simulink model "Test_mcb_pmsm_foc_sim_RL"  (R2020b)
settings: Solver=FixedStepDiscrete  StartTime=0.0  StopTime=6  RelTol=1e-3  EnableMultiTasking=on
values from neighbouring files (symbols this model uses):
  coeff_d = readmatrix('C:\Users\terzo\LearningX\advanced_ML\model_tree\output_d\coeff.txt')    [readtrees.m]
  coeff_q = readmatrix('C:\Users\terzo\LearningX\advanced_ML\model_tree\output_q\coeff.txt')    [readtrees.m]
  index_d = readmatrix('C:\Users\terzo\LearningX\advanced_ML\model_tree\output_d\index.txt')    [readtrees.m]
  index_q = readmatrix('C:\Users\terzo\LearningX\advanced_ML\model_tree\output_q\index.txt')    [readtrees.m]
  intercept_d = readmatrix('C:\Users\terzo\LearningX\advanced_ML\model_tree\output_d\intercept.txt')    [readtrees.m]
  intercept_q = readmatrix('C:\Users\terzo\LearningX\advanced_ML\model_tree\output_q\intercept.txt')    [readtrees.m]
  inverter = mcb_SetInverterParameters_RL('BoostXL-DRV8305')    [sim_data.m]
  maxAngleIn = 1    [sim_data.m]
  MechOfstInputType = pmsm.p    [sim_data.m]
  PI_params = mcb.internal.SetControllerParameters(pmsm,inverter,PU_System,T_pwm,Ts,Ts_speed)    [sim_data.m]
  PU_System = mcb_SetPUSystem_RL(pmsm,inverter)    [sim_data.m]
  threshold_d = readmatrix('C:\Users\terzo\LearningX\advanced_ML\model_tree\output_d\treshold.txt')    [readtrees.m]
  threshold_q = readmatrix('C:\Users\terzo\LearningX\advanced_ML\model_tree\output_q\treshold.txt')    [readtrees.m]
  Ts_motor = T_pwm/2    (= 0.0001)    [sim_data.m]
  Ts_simulink = T_pwm/2    (= 0.0001)    [sim_data.m]
  Ts_speed = 10*Ts    (= 0.002)    [sim_data.m]
undefined symbols (not defined in the file or in its folder): DiscIntNeverNeededParam, pmsm
libraries: mcbcontrolslib x22, mcbpositiondecoderlib x6, simulink x4, mcbplantlib x2, autolibpmsmexterior x2, rllib x1
(part 1 of 2)
settings Model: ExtModeTrigDuration=8  Creator=The MathWorks, Inc.  LastModifiedBy=terzo
settings DataIOCC: DSMLogging=off  InspectSignalLogs=on
settings OptimizationCC: DefaultParameterBehavior=Inlined  DefaultUnderspecifiedDataType=single  EnhancedBackFolding=on  PassReuseOutputArgsAs=Individual arguments  ZeroExternalMemoryAtStartup=off  ZeroInternalMemoryAtStartup=off  MaxStackSize=1024  OptimizeBlockOrder=speed  DifferentSizesBufferReuse=on  OptimizationCustomize=off  DenormalBehavior=FlushToZero  EfficientTunableParamExpr=on
settings DebuggingCC: ParameterPrecisionLossMsg=none  ParameterTunabilityLossMsg=error
settings SFSimCC: MATLABDynamicMemAlloc=off  SimTargetLang=C++
settings RTWCC: Description=Embedded Coder  SystemTargetFile=ert.tlc  TemplateMakefile=ert_default_tmf  Toolchain=Texas Instruments Code Composer Studio (C2000)  TargetLang=C++
settings CodeAppCC: ForceParamTrailComments=on  IgnoreCustomStorageClasses=off  OperatorAnnotations=on  SimulinkDataObjDesc=on  SFDataObjDesc=on  InsertBlockDesc=on
settings ERTTargetCC: TargetLangStandard=C++03 (ISO)  CodeReplacementLibrary=TI C28x  CodeInterfacePackaging=C++ class  ExtModeStaticAllocSize=10000  RootIOFormat=Structure reference  ERTCustomFileTemplate=example_file_process.tlc

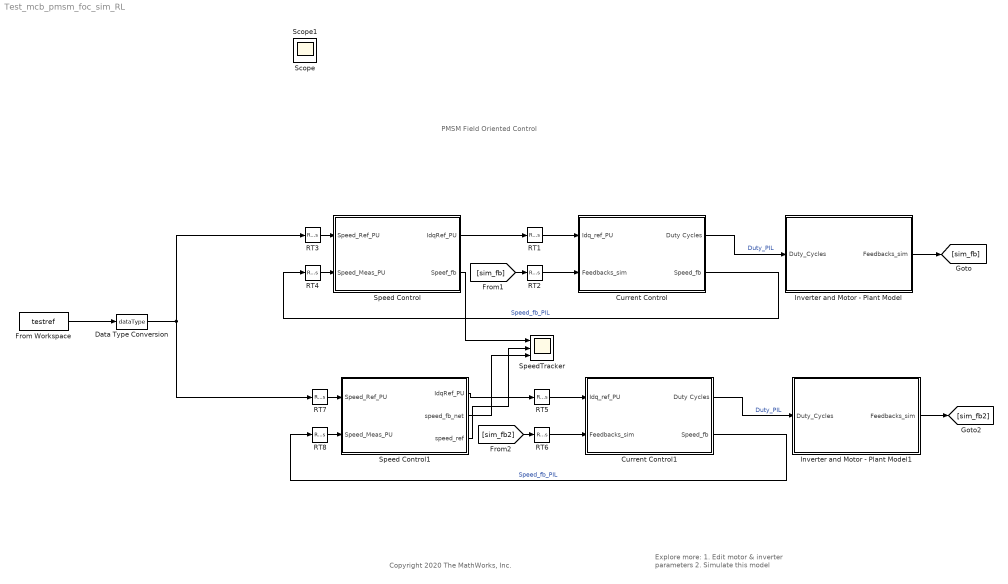
== system Test_mcb_pmsm_foc_sim_RL ==
  note: Explore more:
      | 1. Edit motor & inverter parameters
      | 2. Simulate this model
  note: PMSM Field Oriented Control
  note: Copyright 2020 The MathWorks, Inc.
  Current Control : Subsystem  TreatAsAtomicUnit=on
  Current Control1 : Subsystem  TreatAsAtomicUnit=on
  Data Type Conversion : DataTypeConversion  OutDataTypeStr=dataType
  From Workspace : FromWorkspace  VariableName=testref  SampleTime=Ts_speed
  Inverter and Motor - Plant Model : Subsystem
  Inverter and Motor - Plant Model1 : Subsystem
  RT{1..2,5..6} (4 alike) : RateTransition  Integrity=off  Deterministic=off  OutPortSampleTime=Ts
  RT{3..4,7..8} (4 alike) : RateTransition  Integrity=off  Deterministic=off  OutPortSampleTime=Ts_speed
  Speed Control : Subsystem  TreatAsAtomicUnit=on  SystemSampleTime=Ts_speed
  Speed Control1 : Subsystem  TreatAsAtomicUnit=on  SystemSampleTime=Ts_speed
  SpeedTracker : Scope  NumInputPorts=3
  Scope : Scope
  Scope1 : Scope
  wires:
  RT1/1 -> Current Control/1(Idq_ref_PU)
  Current Control/1(Duty Cycles) -> Inverter and Motor - Plant Model/1(Duty_Cycles)  "Duty_PIL"
  RT4/1 -> Speed Control/2(Speed_Meas_PU)
  Current Control/2(Speed_fb) -> RT4/1  "Speed_fb_PIL"
  [sim_fb] -> RT2/1
  Inverter and Motor - Plant Model/1(Feedbacks_sim) -> [sim_fb]
  RT3/1 -> Speed Control/1(Speed_Ref_PU)
  RT2/1 -> Current Control/2(Feedbacks_sim)
  Speed Control/1(IdqRef_PU) -> RT1/1
  From Workspace/1 -> Data Type Conversion/1
  RT7/1 -> Speed Control1/1(Speed_Ref_PU)
  Inverter and Motor - Plant Model1/1(Feedbacks_sim) -> [sim_fb2]
  RT6/1 -> Current Control1/2(Feedbacks_sim)
  Current Control1/1(Duty Cycles) -> Inverter and Motor - Plant Model1/1(Duty_Cycles)  "Duty_PIL"
  Speed Control1/1(IdqRef_PU) -> RT5/1
  Data Type Conversion/1 -> RT7/1, RT3/1
  RT5/1 -> Current Control1/1(Idq_ref_PU)
  [sim_fb2] -> RT6/1
  Current Control1/2(Speed_fb) -> RT8/1  "Speed_fb_PIL"
  RT8/1 -> Speed Control1/2(Speed_Meas_PU)
  Speed Control/2(Speef_fb) -> SpeedTracker/1
  Speed Control1/2(speed_fb_net) -> SpeedTracker/3
  Speed Control1/3(speed_ref) -> SpeedTracker/2

== system Test_mcb_pmsm_foc_sim_RL/Current Control ==
  Idq_ref_PU : Inport
  Feedbacks_sim : Inport  Port=2
  Control_System : Subsystem
  Demux1 : Demux
  Input Scaling : Subsystem
  Duty Cycles : Outport  InitialOutput=0  VectorParamsAs1DForOutWhenUnconnected=off
  Speed_fb : Outport  Port=2  InitialOutput=0  VectorParamsAs1DForOutWhenUnconnected=off
  wires:
  Input Scaling/2(Pos_PU) -> Control_System/2(Pos_PU)  "Pos_PU"
  Input Scaling/3(speed_PU) -> Speed_fb/1  "Speed_PU"
  Input Scaling/1(Iab_meas_PU) -> Control_System/1(Iab_meas_PU)  "Iab_fb_PU"
  Demux1/1 -> Input Scaling/1(Ia_ADC)
  Demux1/2 -> Input Scaling/2(Ib_ADC)
  Demux1/3 -> Input Scaling/3(QEP_Position_Count)
  Demux1/4 -> Input Scaling/4(QEP_Index_Latch)
  Control_System/1(Duty_Cycles) -> Duty Cycles/1
  Feedbacks_sim/1 -> Demux1/1
  Idq_ref_PU/1 -> Control_System/3(Idq_ref_PU)

== system Test_mcb_pmsm_foc_sim_RL/Current Control1 ==
  Idq_ref_PU : Inport
  Feedbacks_sim : Inport  Port=2
  Control_System : Subsystem
  Demux1 : Demux
  Input Scaling : Subsystem
  Duty Cycles : Outport  InitialOutput=0  VectorParamsAs1DForOutWhenUnconnected=off
  Speed_fb : Outport  Port=2  InitialOutput=0  VectorParamsAs1DForOutWhenUnconnected=off
  wires:
  Input Scaling/2(Pos_PU) -> Control_System/2(Pos_PU)  "Pos_PU"
  Input Scaling/3(speed_PU) -> Speed_fb/1  "Speed_PU"
  Input Scaling/1(Iab_meas_PU) -> Control_System/1(Iab_meas_PU)  "Iab_fb_PU"
  Demux1/1 -> Input Scaling/1(Ia_ADC)
  Demux1/2 -> Input Scaling/2(Ib_ADC)
  Demux1/3 -> Input Scaling/3(QEP_Position_Count)
  Demux1/4 -> Input Scaling/4(QEP_Index_Latch)
  Control_System/1(Duty_Cycles) -> Duty Cycles/1
  Feedbacks_sim/1 -> Demux1/1
  Idq_ref_PU/1 -> Control_System/3(Idq_ref_PU)

== system Test_mcb_pmsm_foc_sim_RL/Inverter and Motor - Plant Model ==
  Duty_Cycles : Inport
  Average Inverter : Subsystem
  Load_Profile (Torque) : Subsystem
  RT1 : RateTransition  Deterministic=off  OutPortSampleTime=Ts_simulink
  RT3 : RateTransition  Deterministic=off  OutPortSampleTime=Ts_simulink
  Rate Transition : RateTransition  Deterministic=off  OutPortSampleTime=Ts_motor
  Rate Transition1 : RateTransition  Deterministic=off  OutPortSampleTime=Ts_motor
  Sensor_Measurements : Subsystem
  Surface Mount PMSM : autolibpmsmexterior/Surface Mount PMSM  port_config=Torque  sim_type=Discrete  Ts=Ts_motor  FilePath=E:\Sandbox\Bauto\Work\surfacepmsm_motordata.m  P=pmsm.p  Rs=pmsm.Rs  Ldq_=pmsm.Ld  KConstText=Permanent flux linkage constant (lambda_pm):  lambda_pm=pmsm.FluxPM  Ke=159.9771  Kt=1.323  mechanical=[pmsm.J, pmsm.B, 0]  idq0=[0 0]  theta_init=0  omega_init=0  KConst=pmsm.FluxPM  lambda_pm_calc=pmsm.FluxPM  RefBlkName='autolibpmsmexterior/Surface Mount PMSM'  aMode=5  Ldq="[0.0002      0.0002]"
      settings: SourceProductBaseCode=PW,MT,UV,VE,VP
  Terminator : Terminator
  Feedbacks_sim : Outport  VectorParamsAs1DForOutWhenUnconnected=off
  wires:
  Surface Mount PMSM/1 -> RT3/1
  RT1/1 -> Sensor_Measurements/2(PhaseCurr)
  RT3/1 -> Sensor_Measurements/1(Info)
  Average Inverter/1(Vabc) -> Rate Transition/1
  Rate Transition/1 -> Surface Mount PMSM/2
  Surface Mount PMSM/3 -> Terminator/1
  Rate Transition1/1 -> Surface Mount PMSM/1
  Sensor_Measurements/1(Sim_fb) -> Feedbacks_sim/1
  Surface Mount PMSM/2 -> RT1/1  "Iabc"
  Load_Profile (Torque)/1(Load_Trq) -> Rate Transition1/1
  Duty_Cycles/1 -> Average Inverter/1(Duty_abc)

== system Test_mcb_pmsm_foc_sim_RL/Inverter and Motor - Plant Model1 ==
  Duty_Cycles : Inport
  Average Inverter : Subsystem
  Load_Profile (Torque) : Subsystem
  RT1 : RateTransition  Deterministic=off  OutPortSampleTime=Ts_simulink
  RT3 : RateTransition  Deterministic=off  OutPortSampleTime=Ts_simulink
  Rate Transition : RateTransition  Deterministic=off  OutPortSampleTime=Ts_motor
  Rate Transition1 : RateTransition  Deterministic=off  OutPortSampleTime=Ts_motor
  Sensor_Measurements : Subsystem
  Surface Mount PMSM : autolibpmsmexterior/Surface Mount PMSM  port_config=Torque  sim_type=Discrete  Ts=Ts_motor  FilePath=E:\Sandbox\Bauto\Work\surfacepmsm_motordata.m  P=pmsm.p  Rs=pmsm.Rs  Ldq_=pmsm.Ld  KConstText=Permanent flux linkage constant (lambda_pm):  lambda_pm=pmsm.FluxPM  Ke=159.9771  Kt=1.323  mechanical=[pmsm.J, pmsm.B, 0]  idq0=[0 0]  theta_init=0  omega_init=0  KConst=pmsm.FluxPM  lambda_pm_calc=pmsm.FluxPM  RefBlkName='autolibpmsmexterior/Surface Mount PMSM'  aMode=5  Ldq="[0.0002      0.0002]"
      settings: SourceProductBaseCode=PW,MT,UV,VE,VP
  Terminator : Terminator
  Feedbacks_sim : Outport  VectorParamsAs1DForOutWhenUnconnected=off
  wires:
  Surface Mount PMSM/1 -> RT3/1
  RT1/1 -> Sensor_Measurements/2(PhaseCurr)
  RT3/1 -> Sensor_Measurements/1(Info)
  Average Inverter/1(Vabc) -> Rate Transition/1
  Rate Transition/1 -> Surface Mount PMSM/2
  Surface Mount PMSM/3 -> Terminator/1
  Rate Transition1/1 -> Surface Mount PMSM/1
  Sensor_Measurements/1(Sim_fb) -> Feedbacks_sim/1
  Surface Mount PMSM/2 -> RT1/1  "Iabc"
  Load_Profile (Torque)/1(Load_Trq) -> Rate Transition1/1
  Duty_Cycles/1 -> Average Inverter/1(Duty_abc)

== system Test_mcb_pmsm_foc_sim_RL/Speed Control ==
  Speed_Ref_PU : Inport
  Speed_Meas_PU : Inport  Port=2
  Gain3 : Gain  Gain=pmsm.N_base
  IIR Filter : mcbcontrolslib/IIR Filter  Filter_constant=0.1
      settings: SourceProductBaseCode=MT
  Id_ref : Constant  Value=0  OutDataTypeStr=dataType  SampleTime=Ts_speed
  Mux1 : Mux  Inputs=2
  PI_Controller_Speed : Subsystem
  IdqRef_PU : Outport  VectorParamsAs1DForOutWhenUnconnected=off
  Speef_fb : Outport  Port=2
  wires:
  Speed_Meas_PU/1 -> Gain3/1, PI_Controller_Speed/2(N_fb)  "Speed_fb"
  Id_ref/1 -> Mux1/1
  PI_Controller_Speed/1(Iq_ref) -> Mux1/2
  Mux1/1 -> IdqRef_PU/1
  Speed_Ref_PU/1 -> IIR Filter/1  "Speed_Ref"
  IIR Filter/1 -> PI_Controller_Speed/1(N_ref)  "Speed_Ref"
  Gain3/1 -> Speef_fb/1  "speed_fb_rpm"

== system Test_mcb_pmsm_foc_sim_RL/Speed Control1 ==
  Speed_Ref_PU : Inport
  Speed_Meas_PU : Inport  Port=2
  Gain1 : Gain  Gain=pmsm.N_base
  Gain3 : Gain  Gain=pmsm.N_base
  IIR Filter : mcbcontrolslib/IIR Filter  Filter_constant=0.1
      settings: SourceProductBaseCode=MT
  Id_ref : Constant  Value=0  OutDataTypeStr=dataType  SampleTime=Ts_speed
  Mux1 : Mux  Inputs=2
  PI_Controller_Speed : Subsystem
  IdqRef_PU : Outport  VectorParamsAs1DForOutWhenUnconnected=off
  speed_fb_net : Outport  Port=2
  speed_ref : Outport  Port=3
  wires:
  Speed_Meas_PU/1 -> Gain3/1, PI_Controller_Speed/2(N_fb)  "Speed_fb"
  Id_ref/1 -> Mux1/1
  PI_Controller_Speed/1(Iq_ref) -> Mux1/2
  Mux1/1 -> IdqRef_PU/1
  Speed_Ref_PU/1 -> IIR Filter/1  "Speed_Ref"
  IIR Filter/1 -> Gain1/1, PI_Controller_Speed/1(N_ref)  "Speed_Ref"
  Gain3/1 -> speed_fb_net/1  "speed_fb_net_rpm"
  Gain1/1 -> speed_ref/1  "speed_ref_rpm"

== system Test_mcb_pmsm_foc_sim_RL/Current Control/Control_System ==
  Iab_meas_PU : Inport
  Pos_PU : Inport  Port=2
  Idq_ref_PU : Inport  Port=3
  Closed Loop Control : Subsystem
  Duty_Cycles : Outport  VectorParamsAs1DForOutWhenUnconnected=off
  wires:
  Iab_meas_PU/1 -> Closed Loop Control/1(Iab_meas_PU)
  Pos_PU/1 -> Closed Loop Control/2(Pos_PU)
  Idq_ref_PU/1 -> Closed Loop Control/3(Idq_ref_PU)
  Closed Loop Control/1(Vabc in PU) -> Duty_Cycles/1

== system Test_mcb_pmsm_foc_sim_RL/Current Control/Input Scaling ==
  note: Current Measurements
  note: Position & Speed Measurements
  note: QEP
  Ia_ADC : Inport
  Ib_ADC : Inport  Port=2
  QEP_Position_Count : Inport  Port=3
  QEP_Index_Latch : Inport  Port=4
  " Calculate Position and Speed" : Subsystem
  Calculate Phase Currents : Subsystem
  IndexOffset : Constant  Value=pmsm.PositionOffset  OutDataTypeStr=dataType  SampleTime=-1
  Iab_meas_PU : Outport
  Pos_PU : Outport  Port=2
  speed_PU : Outport  Port=3
  wires:
  " Calculate Position and Speed"/2(speed) -> speed_PU/1
  Calculate Phase Currents/1(Iab_meas_PU) -> Iab_meas_PU/1  "Iab_fb_PU"
  QEP_Position_Count/1 -> " Calculate Position and Speed"/1(QEP_Position_Count)
  " Calculate Position and Speed"/1(Theta_e) -> Pos_PU/1
  Ia_ADC/1 -> Calculate Phase Currents/1(Ia_ADC)
  Ib_ADC/1 -> Calculate Phase Currents/2(Ib_ADC)
  QEP_Index_Latch/1 -> " Calculate Position and Speed"/2(QEP_Index_Latch)
  IndexOffset/1 -> " Calculate Position and Speed"/3(Offset)

== system Test_mcb_pmsm_foc_sim_RL/Current Control1/Control_System ==
  Iab_meas_PU : Inport
  Pos_PU : Inport  Port=2
  Idq_ref_PU : Inport  Port=3
  Closed Loop Control : Subsystem
  Duty_Cycles : Outport  VectorParamsAs1DForOutWhenUnconnected=off
  wires:
  Iab_meas_PU/1 -> Closed Loop Control/1(Iab_meas_PU)
  Pos_PU/1 -> Closed Loop Control/2(Pos_PU)
  Idq_ref_PU/1 -> Closed Loop Control/3(Idq_ref_PU)
  Closed Loop Control/1(Vabc in PU) -> Duty_Cycles/1

== system Test_mcb_pmsm_foc_sim_RL/Current Control1/Input Scaling ==
  note: Current Measurements
  note: Position & Speed Measurements
  note: QEP
  Ia_ADC : Inport
  Ib_ADC : Inport  Port=2
  QEP_Position_Count : Inport  Port=3
  QEP_Index_Latch : Inport  Port=4
  " Calculate Position and Speed" : Subsystem
  Calculate Phase Currents : Subsystem
  IndexOffset : Constant  Value=pmsm.PositionOffset  OutDataTypeStr=dataType  SampleTime=-1
  Iab_meas_PU : Outport
  Pos_PU : Outport  Port=2
  speed_PU : Outport  Port=3
  wires:
  " Calculate Position and Speed"/2(speed) -> speed_PU/1
  Calculate Phase Currents/1(Iab_meas_PU) -> Iab_meas_PU/1  "Iab_fb_PU"
  QEP_Position_Count/1 -> " Calculate Position and Speed"/1(QEP_Position_Count)
  " Calculate Position and Speed"/1(Theta_e) -> Pos_PU/1
  Ia_ADC/1 -> Calculate Phase Currents/1(Ia_ADC)
  Ib_ADC/1 -> Calculate Phase Currents/2(Ib_ADC)
  QEP_Index_Latch/1 -> " Calculate Position and Speed"/2(QEP_Index_Latch)
  IndexOffset/1 -> " Calculate Position and Speed"/3(Offset)

== system Test_mcb_pmsm_foc_sim_RL/Inverter and Motor - Plant Model/Average Inverter ==
  Duty_abc : Inport
  Average-Value Inverter : mcbplantlib/Average-Value Inverter
  Constant2 : Constant  Value=inverter.V_dc  OutDataTypeStr=single  SampleTime=-1
  Data Type Conversion1 : DataTypeConversion  OutDataTypeStr=single  RndMeth=Simplest
  Rate Transition3 : RateTransition  Deterministic=off  OutPortSampleTime=Ts_inverter
  Vabc : Outport  VectorParamsAs1DForOutWhenUnconnected=off
  wires:
  Constant2/1 -> Average-Value Inverter/2
  Data Type Conversion1/1 -> Rate Transition3/1
  Duty_abc/1 -> Data Type Conversion1/1
  Rate Transition3/1 -> Average-Value Inverter/1
  Average-Value Inverter/1 -> Vabc/1

== system Test_mcb_pmsm_foc_sim_RL/Inverter and Motor - Plant Model/Load_Profile (Torque) ==
  Data Type Conversion : DataTypeConversion  OutDataTypeStr=single
  IIR Filter : mcbcontrolslib/IIR Filter  Filter_constant=0.01
      settings: SourceProductBaseCode=MT
  T_load : Step  Time=100  After=0  SampleTime=Ts_simulink
  T_load1 : Step  Commented=on  Time=0.8  Before=0.05*pmsm.T_rated  After=0.05*pmsm.T_rated  SampleTime=Ts_simulink
  Load_Trq : Outport  VectorParamsAs1DForOutWhenUnconnected=off
  wires:
  Data Type Conversion/1 -> IIR Filter/1
  IIR Filter/1 -> Load_Trq/1
  T_load/1 -> Data Type Conversion/1

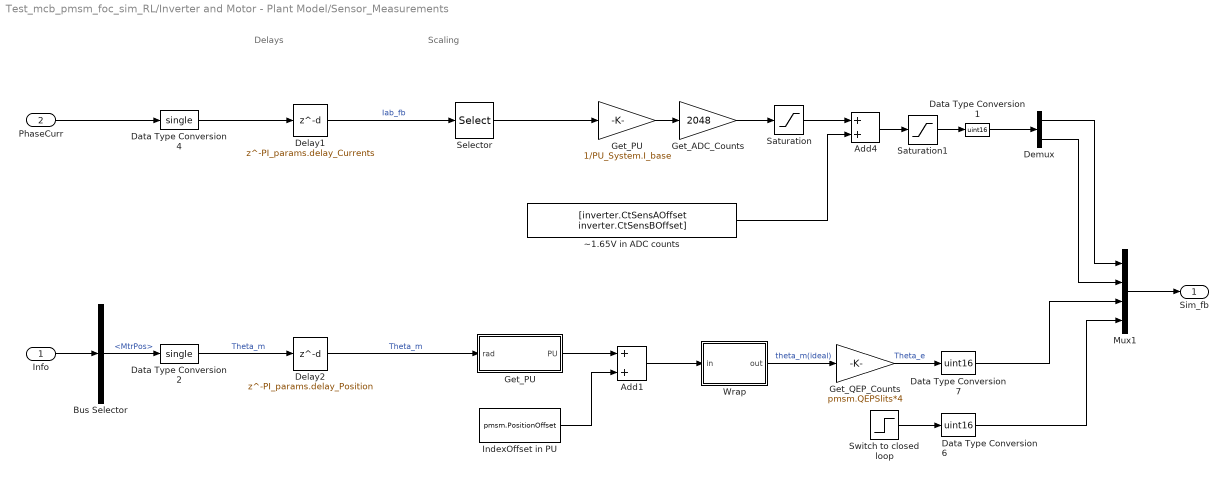
== system Test_mcb_pmsm_foc_sim_RL/Inverter and Motor - Plant Model/Sensor_Measurements ==
  note: Scaling
  note: Delays
  Info : Inport
  PhaseCurr : Inport  Port=2
  Add1 : Sum  RndMeth=Simplest
  Add4 : Sum  OutDataTypeStr=uint16
  Bus Selector : BusSelector  OutputSignals=MtrPos
  Data Type Conversion1 : DataTypeConversion  OutDataTypeStr=uint16
  Data Type Conversion2 : DataTypeConversion  OutDataTypeStr=single  RndMeth=Simplest
  Data Type Conversion4 : DataTypeConversion  OutDataTypeStr=single  RndMeth=Simplest
  Data Type Conversion6 : DataTypeConversion  OutDataTypeStr=uint16  RndMeth=Simplest
  Data Type Conversion7 : DataTypeConversion  OutDataTypeStr=uint16  RndMeth=Simplest
  Delay1 : Delay  DelayLength=PI_params.delay_Currents
  Delay2 : Delay  DelayLength=PI_params.delay_Position
  Demux : Demux  Outputs=2
  Get_ADC_Counts : Gain  Gain=2048  RndMeth=Simplest  OutDataTypeStr=Inherit: Same as input
  Get_PU : Gain  Gain=1/PU_System.I_base  RndMeth=Simplest
  "Get_PU " : Subsystem
  Get_QEP_Counts : Gain  Gain=pmsm.QEPSlits*4  OutDataTypeStr=uint16  RndMeth=Simplest
  IndexOffset in PU : Constant  Value=pmsm.PositionOffset  OutDataTypeStr=single  SampleTime=-1
  Mux1 : Mux
  Saturation : Saturate  UpperLimit=2048  LowerLimit=-2048
  Saturation1 : Saturate  UpperLimit=4095  LowerLimit=0
  Selector : Selector  InputPortWidth=3  IndexOptions=Index vector (dialog)  Indices=[1 2]  OutputSizes=1
  "Switch to closed loop " : Step  Time=0.1  SampleTime=Ts_motor
  Wrap : Subsystem
  ~1.65V in ADC counts : Constant  Value=[inverter.CtSensAOffset inverter.CtSensBOffset]  OutDataTypeStr=uint16  SampleTime=-1
  Sim_fb : Outport  VectorParamsAs1DForOutWhenUnconnected=off
  wires:
  Get_ADC_Counts/1 -> Saturation/1
  Saturation1/1 -> Data Type Conversion1/1
  Add4/1 -> Saturation1/1
  Data Type Conversion1/1 -> Demux/1
  ~1.65V in ADC counts/1 -> Add4/2
  Delay1/1 -> Selector/1  "Iab_fb"
  Saturation/1 -> Add4/1
  Data Type Conversion4/1 -> Delay1/1
  Selector/1 -> Get_PU/1
  PhaseCurr/1 -> Data Type Conversion4/1
  Get_PU/1 -> Get_ADC_Counts/1
  Info/1 -> Bus Selector/1
  Bus Selector/1 -> Data Type Conversion2/1  "<MtrPos>"
  Demux/1 -> Mux1/1
  Mux1/1 -> Sim_fb/1
  Demux/2 -> Mux1/2
  Data Type Conversion2/1 -> Delay2/1  "Theta_m"
  Add1/1 -> Wrap/1(in)
  Delay2/1 -> "Get_PU "/1(rad)  "Theta_m"
  Wrap/1(out) -> Get_QEP_Counts/1  "theta_m(ideal)"
  "Get_PU "/1(PU) -> Add1/1
  Get_QEP_Counts/1 -> Data Type Conversion7/1  "Theta_e"
  IndexOffset in PU/1 -> Add1/2
  Data Type Conversion7/1 -> Mux1/3
  Data Type Conversion6/1 -> Mux1/4
  "Switch to closed loop "/1 -> Data Type Conversion6/1

== system Test_mcb_pmsm_foc_sim_RL/Inverter and Motor - Plant Model1/Average Inverter ==
  Duty_abc : Inport
  Average-Value Inverter : mcbplantlib/Average-Value Inverter
  Constant2 : Constant  Value=inverter.V_dc  OutDataTypeStr=single  SampleTime=-1
  Data Type Conversion1 : DataTypeConversion  OutDataTypeStr=single  RndMeth=Simplest
  Rate Transition3 : RateTransition  Deterministic=off  OutPortSampleTime=Ts_inverter
  Vabc : Outport  VectorParamsAs1DForOutWhenUnconnected=off
  wires:
  Constant2/1 -> Average-Value Inverter/2
  Data Type Conversion1/1 -> Rate Transition3/1
  Duty_abc/1 -> Data Type Conversion1/1
  Rate Transition3/1 -> Average-Value Inverter/1
  Average-Value Inverter/1 -> Vabc/1

== system Test_mcb_pmsm_foc_sim_RL/Inverter and Motor - Plant Model1/Load_Profile (Torque) ==
  Data Type Conversion : DataTypeConversion  OutDataTypeStr=single
  IIR Filter : mcbcontrolslib/IIR Filter  Filter_constant=0.01
      settings: SourceProductBaseCode=MT
  T_load : Step  Time=100  After=0  SampleTime=Ts_simulink
  T_load1 : Step  Commented=on  Time=0.8  Before=0.05*pmsm.T_rated  After=0.05*pmsm.T_rated  SampleTime=Ts_simulink
  Load_Trq : Outport  VectorParamsAs1DForOutWhenUnconnected=off
  wires:
  Data Type Conversion/1 -> IIR Filter/1
  IIR Filter/1 -> Load_Trq/1
  T_load/1 -> Data Type Conversion/1

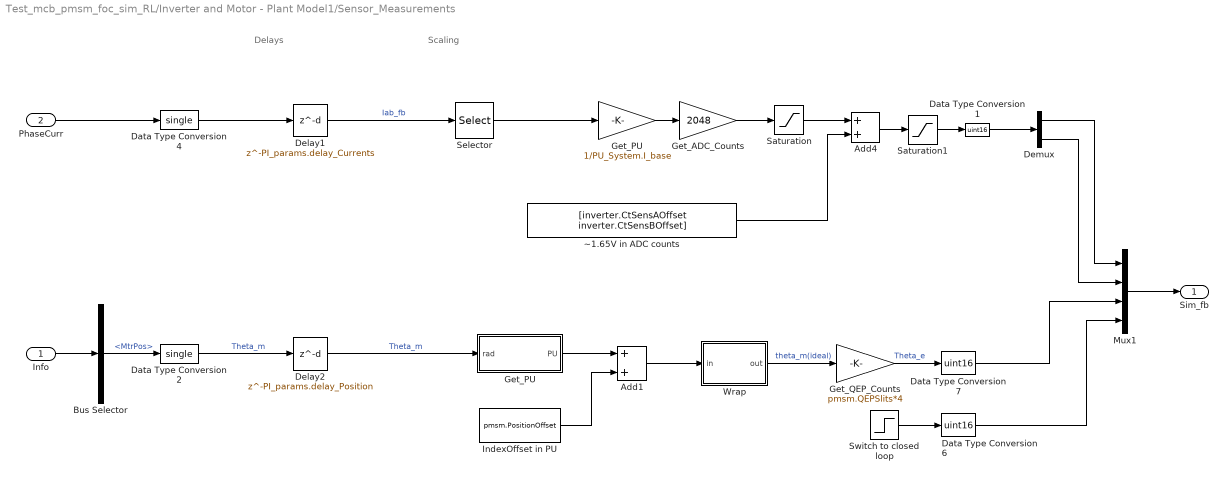
== system Test_mcb_pmsm_foc_sim_RL/Inverter and Motor - Plant Model1/Sensor_Measurements ==
  note: Scaling
  note: Delays
  Info : Inport
  PhaseCurr : Inport  Port=2
  Add1 : Sum  RndMeth=Simplest
  Add4 : Sum  OutDataTypeStr=uint16
  Bus Selector : BusSelector  OutputSignals=MtrPos
  Data Type Conversion1 : DataTypeConversion  OutDataTypeStr=uint16
  Data Type Conversion2 : DataTypeConversion  OutDataTypeStr=single  RndMeth=Simplest
  Data Type Conversion4 : DataTypeConversion  OutDataTypeStr=single  RndMeth=Simplest
  Data Type Conversion6 : DataTypeConversion  OutDataTypeStr=uint16  RndMeth=Simplest
  Data Type Conversion7 : DataTypeConversion  OutDataTypeStr=uint16  RndMeth=Simplest
  Delay1 : Delay  DelayLength=PI_params.delay_Currents
  Delay2 : Delay  DelayLength=PI_params.delay_Position
  Demux : Demux  Outputs=2
  Get_ADC_Counts : Gain  Gain=2048  RndMeth=Simplest  OutDataTypeStr=Inherit: Same as input
  Get_PU : Gain  Gain=1/PU_System.I_base  RndMeth=Simplest
  "Get_PU " : Subsystem
  Get_QEP_Counts : Gain  Gain=pmsm.QEPSlits*4  OutDataTypeStr=uint16  RndMeth=Simplest
  IndexOffset in PU : Constant  Value=pmsm.PositionOffset  OutDataTypeStr=single  SampleTime=-1
  Mux1 : Mux
  Saturation : Saturate  UpperLimit=2048  LowerLimit=-2048
  Saturation1 : Saturate  UpperLimit=4095  LowerLimit=0
  Selector : Selector  InputPortWidth=3  IndexOptions=Index vector (dialog)  Indices=[1 2]  OutputSizes=1
  "Switch to closed loop " : Step  Time=0.1  SampleTime=Ts_motor
  Wrap : Subsystem
  ~1.65V in ADC counts : Constant  Value=[inverter.CtSensAOffset inverter.CtSensBOffset]  OutDataTypeStr=uint16  SampleTime=-1
  Sim_fb : Outport  VectorParamsAs1DForOutWhenUnconnected=off
  wires:
  Get_ADC_Counts/1 -> Saturation/1
  Saturation1/1 -> Data Type Conversion1/1
  Add4/1 -> Saturation1/1
  Data Type Conversion1/1 -> Demux/1
  ~1.65V in ADC counts/1 -> Add4/2
  Delay1/1 -> Selector/1  "Iab_fb"
  Saturation/1 -> Add4/1
  Data Type Conversion4/1 -> Delay1/1
  Selector/1 -> Get_PU/1
  PhaseCurr/1 -> Data Type Conversion4/1
  Get_PU/1 -> Get_ADC_Counts/1
  Info/1 -> Bus Selector/1
  Bus Selector/1 -> Data Type Conversion2/1  "<MtrPos>"
  Demux/1 -> Mux1/1
  Mux1/1 -> Sim_fb/1
  Demux/2 -> Mux1/2
  Data Type Conversion2/1 -> Delay2/1  "Theta_m"
  Add1/1 -> Wrap/1(in)
  Delay2/1 -> "Get_PU "/1(rad)  "Theta_m"
  Wrap/1(out) -> Get_QEP_Counts/1  "theta_m(ideal)"
  "Get_PU "/1(PU) -> Add1/1
  Get_QEP_Counts/1 -> Data Type Conversion7/1  "Theta_e"
  IndexOffset in PU/1 -> Add1/2
  Data Type Conversion7/1 -> Mux1/3
  Data Type Conversion6/1 -> Mux1/4
  "Switch to closed loop "/1 -> Data Type Conversion6/1

== system Test_mcb_pmsm_foc_sim_RL/Speed Control/PI_Controller_Speed ==
  N_ref : Inport
  N_fb : Inport  Port=2
  Constant : Constant  OutDataTypeStr=boolean
  Discrete PI Controller with anti-windup & reset : mcbcontrolslib/Discrete PI Controller  with anti-windup & reset  UpperSaturationLimit=1  LowerSaturationLimit=-1
      settings: SourceProductBaseCode=MT
  Ki1 : Constant  Value=PI_params.Ki_speed*Ts_speed  OutDataTypeStr=dataType  SampleTime=-1
  Ki2 : Constant  Value=0  OutDataTypeStr=dataType  SampleTime=-1
  Kp1 : Constant  Value=PI_params.Kp_speed  OutDataTypeStr=dataType  SampleTime=-1
  Logical Operator : Logic  Operator=NOT  IconShape=distinctive  AllPortsSameDT=off  OutDataTypeStr=boolean
  Sum : Sum  Inputs=|+-  OutDataTypeStr=Inherit: Same as first input
  Iq_ref : Outport  VectorParamsAs1DForOutWhenUnconnected=off
  wires:
  Discrete PI Controller with anti-windup & reset/1 -> Iq_ref/1
  Ki1/1 -> Discrete PI Controller with anti-windup & reset/3
  Kp1/1 -> Discrete PI Controller with anti-windup & reset/2
  N_fb/1 -> Sum/2
  N_ref/1 -> Sum/1
  Sum/1 -> Discrete PI Controller with anti-windup & reset/1
  Logical Operator/1 -> Discrete PI Controller with anti-windup & reset/4
  Ki2/1 -> Discrete PI Controller with anti-windup & reset/5
  Constant/1 -> Logical Operator/1

== system Test_mcb_pmsm_foc_sim_RL/Speed Control1/PI_Controller_Speed ==
  N_ref : Inport
  N_fb : Inport  Port=2
  Constant : Constant  OutDataTypeStr=boolean
  Discrete PI Controller with anti-windup & reset : mcbcontrolslib/Discrete PI Controller  with anti-windup & reset  UpperSaturationLimit=1  LowerSaturationLimit=-1
      settings: SourceProductBaseCode=MT
  Ki1 : Constant  Value=PI_params.Ki_speed*Ts_speed  OutDataTypeStr=dataType  SampleTime=-1
  Ki2 : Constant  Value=0  OutDataTypeStr=dataType  SampleTime=-1
  Kp1 : Constant  Value=PI_params.Kp_speed  OutDataTypeStr=dataType  SampleTime=-1
  Logical Operator : Logic  Operator=NOT  IconShape=distinctive  AllPortsSameDT=off  OutDataTypeStr=boolean
  Sum : Sum  Inputs=|+-  OutDataTypeStr=Inherit: Same as first input
  Iq_ref : Outport  VectorParamsAs1DForOutWhenUnconnected=off
  wires:
  Discrete PI Controller with anti-windup & reset/1 -> Iq_ref/1
  Ki1/1 -> Discrete PI Controller with anti-windup & reset/3
  Kp1/1 -> Discrete PI Controller with anti-windup & reset/2
  N_fb/1 -> Sum/2
  N_ref/1 -> Sum/1
  Sum/1 -> Discrete PI Controller with anti-windup & reset/1
  Logical Operator/1 -> Discrete PI Controller with anti-windup & reset/4
  Ki2/1 -> Discrete PI Controller with anti-windup & reset/5
  Constant/1 -> Logical Operator/1

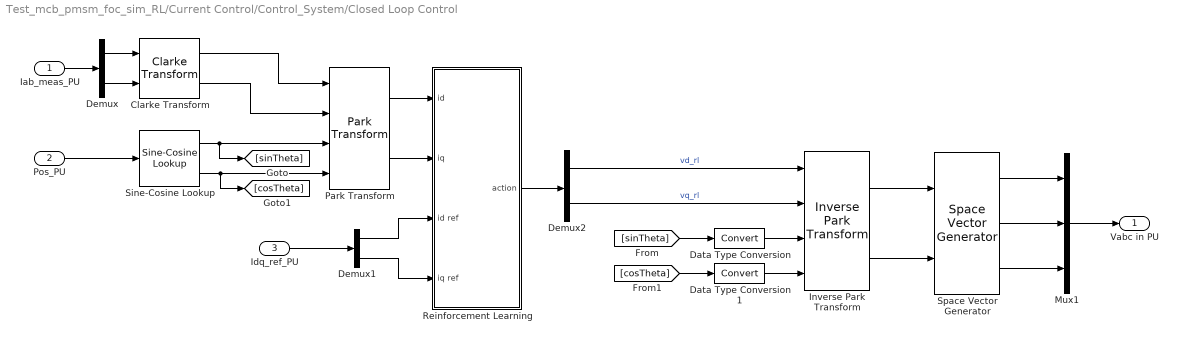
== system Test_mcb_pmsm_foc_sim_RL/Current Control/Control_System/Closed Loop Control ==
  Iab_meas_PU : Inport
  Pos_PU : Inport  Port=2
  Idq_ref_PU : Inport  Port=3
  Clarke Transform : mcbcontrolslib/Clarke Transform  VariantControl=Variant2
  Data Type Conversion : DataTypeConversion
  Data Type Conversion1 : DataTypeConversion
  Demux : Demux  Outputs=2
  Demux1 : Demux  Outputs=2
  Demux2 : Demux  Outputs=2
  Inverse Park Transform : mcbcontrolslib/Inverse Park Transform  AxisAlignment=D-axis
  Mux1 : Mux  Inputs=3
  Park Transform : mcbcontrolslib/Park Transform  AxisAlignment=D-axis
      settings: SourceProductBaseCode=MT
  Reinforcement Learning : Subsystem
  Sine-Cosine Lookup : mcbcontrolslib/Sine-Cosine Lookup  AngleInput=Per-unit  N_points=1024
      settings: SourceProductBaseCode=MT
  Space Vector Generator : mcbcontrolslib/Space Vector Generator
      settings: SourceProductBaseCode=MT
  Vabc in PU : Outport  VectorParamsAs1DForOutWhenUnconnected=off
  wires:
  Sine-Cosine Lookup/1 -> [sinTheta], Park Transform/3
  Clarke Transform/2 -> Park Transform/2
  Demux/2 -> Clarke Transform/2
  Pos_PU/1 -> Sine-Cosine Lookup/1
  Demux/1 -> Clarke Transform/1
  Inverse Park Transform/2 -> Space Vector Generator/2
  Iab_meas_PU/1 -> Demux/1
  Demux2/1 -> Inverse Park Transform/1  "vd_rl"
  Inverse Park Transform/1 -> Space Vector Generator/1
  Sine-Cosine Lookup/2 -> Park Transform/4, [cosTheta]
  Space Vector Generator/3 -> Mux1/3
  Demux2/2 -> Inverse Park Transform/2  "vq_rl"
  Space Vector Generator/1 -> Mux1/1
  Mux1/1 -> Vabc in PU/1
  Clarke Transform/1 -> Park Transform/1
  Space Vector Generator/2 -> Mux1/2
  Park Transform/1 -> Reinforcement Learning/1(id)
  Park Transform/2 -> Reinforcement Learning/2(iq)
  Idq_ref_PU/1 -> Demux1/1
  Demux1/1 -> Reinforcement Learning/3(id ref)
  Demux1/2 -> Reinforcement Learning/4(iq ref)
  Reinforcement Learning/1(action) -> Demux2/1
  [sinTheta] -> Data Type Conversion/1
  [cosTheta] -> Data Type Conversion1/1
  Data Type Conversion/1 -> Inverse Park Transform/3
  Data Type Conversion1/1 -> Inverse Park Transform/4

== system Test_mcb_pmsm_foc_sim_RL/Current Control/Input Scaling/ Calculate Position and Speed ==
  QEP_Position_Count : Inport
  QEP_Index_Latch : Inport  Port=2
  Offset : Inport  Port=3
  IIR Filter : mcbcontrolslib/IIR Filter  Filter_constant=0.01
      settings: SourceProductBaseCode=MT
  Mechanical to Electrical Position : mcbpositiondecoderlib/Mechanical to Electrical Position  Commented=on  NrPP=pmsm.p  selectedRange=Per unit  MechOfstInputType=Input port  mechOffsetIn=0  maxAngleIn=1  InputDataType=dataType  VariantSelect=fixed-point
      settings: SourceProductBaseCode=MT
  Quadrature Decoder : mcbpositiondecoderlib/Quadrature Decoder  EncoderSlitsPerRevolution=pmsm.QEPSlits  EncoderCountsPerSlit=4  CounterSize=16 bits  ExternalIndexCount=on  PositionUnit=Per unit  PositionDataType=dataType
      settings: SourceProductBaseCode=MT
  Speed Measurement : mcbpositiondecoderlib/Speed Measurement  PositionUnit=Per unit  SpeedCalculationMode=Time interval for speed calculation  SampleTimeAsync=Ts  MaximumApplicationSpeed=6000  SpeedResolution=5e-6  DelayLength=20  MaximumMeasurableSpeed=7499  MeasurableSpeedResolution=3.4925e-06  SpeedUnit=Per unit based on dialog  PerUnitSpeed=PU_System.N_base  SpeedDataType=dataType
      settings: SourceProductBaseCode=MT
  fixed-point : Subsystem  VariantControl=fixed-point
  Theta_e : Outport  VectorParamsAs1DForOutWhenUnconnected=off
  speed : Outport  Port=2  VectorParamsAs1DForOutWhenUnconnected=off
  wires:
  Speed Measurement/1 -> IIR Filter/1
  QEP_Position_Count/1 -> Quadrature Decoder/1
  Quadrature Decoder/1 -> fixed-point/1(ϴm), Speed Measurement/1
  Offset/1 -> fixed-point/2(Offset)
  IIR Filter/1 -> speed/1
  QEP_Index_Latch/1 -> Quadrature Decoder/2
  fixed-point/1(ϴe) -> Theta_e/1

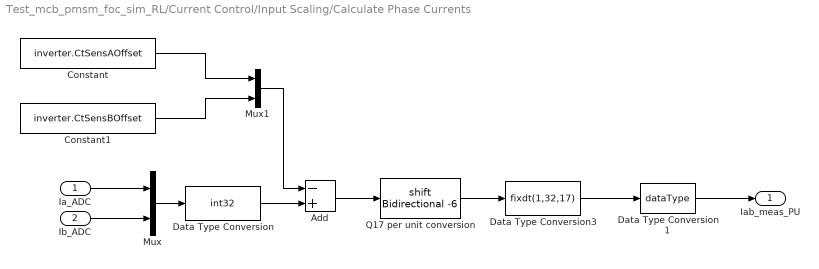
== system Test_mcb_pmsm_foc_sim_RL/Current Control/Input Scaling/Calculate Phase Currents ==
  Ia_ADC : Inport
  Ib_ADC : Inport  Port=2
  Add : Sum  Inputs=-+
  Constant : Constant  Value=inverter.CtSensAOffset  OutDataTypeStr=uint16
  Constant1 : Constant  Value=inverter.CtSensBOffset  OutDataTypeStr=uint16
  Data Type Conversion : DataTypeConversion  OutDataTypeStr=int32  ConvertRealWorld=Stored Integer (SI)  RndMeth=Simplest
  Data Type Conversion1 : DataTypeConversion  OutDataTypeStr=dataType  RndMeth=Simplest
  Data Type Conversion3 : DataTypeConversion  OutDataTypeStr=fixdt(1,32,17)  ConvertRealWorld=Stored Integer (SI)  RndMeth=Simplest
  Mux : Mux  Inputs=2
  Mux1 : Mux  Inputs=2
  Q17 per unit conversion : ArithShift  BitShiftNumber=-6
  Iab_meas_PU : Outport  VectorParamsAs1DForOutWhenUnconnected=off
  wires:
  Q17 per unit conversion/1 -> Data Type Conversion3/1
  Data Type Conversion/1 -> Add/2
  Add/1 -> Q17 per unit conversion/1
  Data Type Conversion3/1 -> Data Type Conversion1/1
  Data Type Conversion1/1 -> Iab_meas_PU/1
  Ia_ADC/1 -> Mux/1
  Ib_ADC/1 -> Mux/2
  Mux/1 -> Data Type Conversion/1
  Constant/1 -> Mux1/1
  Constant1/1 -> Mux1/2
  Mux1/1 -> Add/1

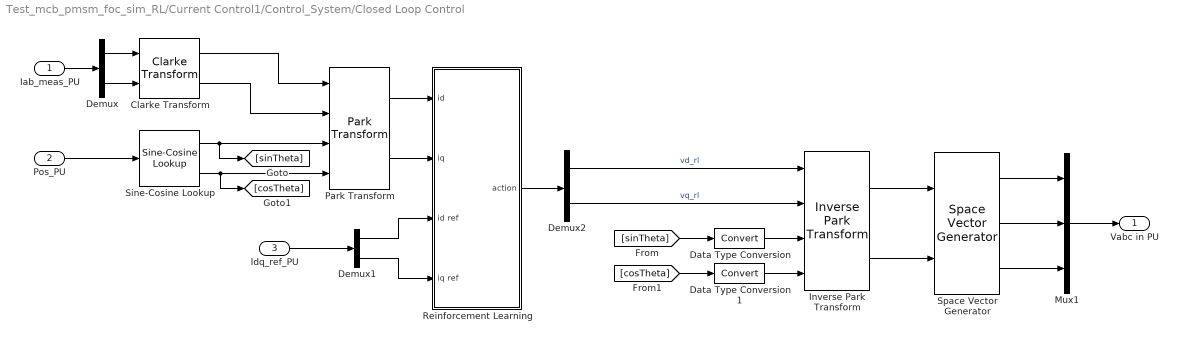
== system Test_mcb_pmsm_foc_sim_RL/Current Control1/Control_System/Closed Loop Control ==
  Iab_meas_PU : Inport
  Pos_PU : Inport  Port=2
  Idq_ref_PU : Inport  Port=3
  Clarke Transform : mcbcontrolslib/Clarke Transform  VariantControl=Variant2
  Data Type Conversion : DataTypeConversion
  Data Type Conversion1 : DataTypeConversion
  Demux : Demux  Outputs=2
  Demux1 : Demux  Outputs=2
  Demux2 : Demux  Outputs=2
  Inverse Park Transform : mcbcontrolslib/Inverse Park Transform  AxisAlignment=D-axis
  Mux1 : Mux  Inputs=3
  Park Transform : mcbcontrolslib/Park Transform  AxisAlignment=D-axis
      settings: SourceProductBaseCode=MT
  Reinforcement Learning : Subsystem
  Sine-Cosine Lookup : mcbcontrolslib/Sine-Cosine Lookup  AngleInput=Per-unit  N_points=1024
      settings: SourceProductBaseCode=MT
  Space Vector Generator : mcbcontrolslib/Space Vector Generator
      settings: SourceProductBaseCode=MT
  Vabc in PU : Outport  VectorParamsAs1DForOutWhenUnconnected=off
  wires:
  Sine-Cosine Lookup/1 -> [sinTheta], Park Transform/3
  Clarke Transform/2 -> Park Transform/2
  Demux/2 -> Clarke Transform/2
  Pos_PU/1 -> Sine-Cosine Lookup/1
  Demux/1 -> Clarke Transform/1
  Inverse Park Transform/2 -> Space Vector Generator/2
  Iab_meas_PU/1 -> Demux/1
  Demux2/1 -> Inverse Park Transform/1  "vd_rl"
  Inverse Park Transform/1 -> Space Vector Generator/1
  Sine-Cosine Lookup/2 -> Park Transform/4, [cosTheta]
  Space Vector Generator/3 -> Mux1/3
  Demux2/2 -> Inverse Park Transform/2  "vq_rl"
  Space Vector Generator/1 -> Mux1/1
  Mux1/1 -> Vabc in PU/1
  Clarke Transform/1 -> Park Transform/1
  Space Vector Generator/2 -> Mux1/2
  Park Transform/1 -> Reinforcement Learning/1(id)
  Park Transform/2 -> Reinforcement Learning/2(iq)
  Idq_ref_PU/1 -> Demux1/1
  Demux1/1 -> Reinforcement Learning/3(id ref)
  Demux1/2 -> Reinforcement Learning/4(iq ref)
  Reinforcement Learning/1(action) -> Demux2/1
  [sinTheta] -> Data Type Conversion/1
  [cosTheta] -> Data Type Conversion1/1
  Data Type Conversion/1 -> Inverse Park Transform/3
  Data Type Conversion1/1 -> Inverse Park Transform/4

== system Test_mcb_pmsm_foc_sim_RL/Current Control1/Input Scaling/ Calculate Position and Speed ==
  QEP_Position_Count : Inport
  QEP_Index_Latch : Inport  Port=2
  Offset : Inport  Port=3
  IIR Filter : mcbcontrolslib/IIR Filter  Filter_constant=0.01
      settings: SourceProductBaseCode=MT
  Mechanical to Electrical Position : mcbpositiondecoderlib/Mechanical to Electrical Position  Commented=on  NrPP=pmsm.p  selectedRange=Per unit  MechOfstInputType=Input port  mechOffsetIn=0  maxAngleIn=1  InputDataType=dataType  VariantSelect=fixed-point
      settings: SourceProductBaseCode=MT
  Quadrature Decoder : mcbpositiondecoderlib/Quadrature Decoder  EncoderSlitsPerRevolution=pmsm.QEPSlits  EncoderCountsPerSlit=4  CounterSize=16 bits  ExternalIndexCount=on  PositionUnit=Per unit  PositionDataType=dataType
      settings: SourceProductBaseCode=MT
  Speed Measurement : mcbpositiondecoderlib/Speed Measurement  PositionUnit=Per unit  SpeedCalculationMode=Time interval for speed calculation  SampleTimeAsync=Ts  MaximumApplicationSpeed=6000  SpeedResolution=5e-6  DelayLength=20  MaximumMeasurableSpeed=7499  MeasurableSpeedResolution=3.4925e-06  SpeedUnit=Per unit based on dialog  PerUnitSpeed=PU_System.N_base  SpeedDataType=dataType
      settings: SourceProductBaseCode=MT
  fixed-point : Subsystem  VariantControl=fixed-point
  Theta_e : Outport  VectorParamsAs1DForOutWhenUnconnected=off
  speed : Outport  Port=2  VectorParamsAs1DForOutWhenUnconnected=off
  wires:
  Speed Measurement/1 -> IIR Filter/1
  QEP_Position_Count/1 -> Quadrature Decoder/1
  Quadrature Decoder/1 -> fixed-point/1(ϴm), Speed Measurement/1
  Offset/1 -> fixed-point/2(Offset)
  IIR Filter/1 -> speed/1
  QEP_Index_Latch/1 -> Quadrature Decoder/2
  fixed-point/1(ϴe) -> Theta_e/1

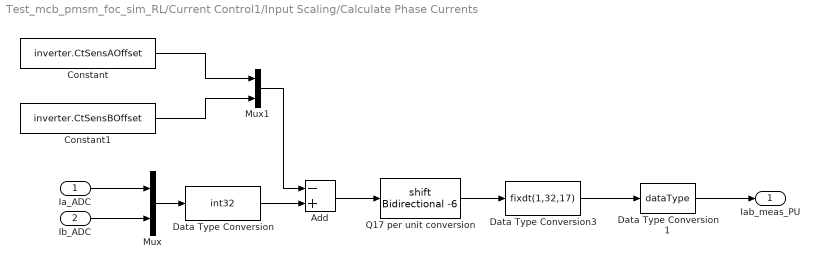
== system Test_mcb_pmsm_foc_sim_RL/Current Control1/Input Scaling/Calculate Phase Currents ==
  Ia_ADC : Inport
  Ib_ADC : Inport  Port=2
  Add : Sum  Inputs=-+
  Constant : Constant  Value=inverter.CtSensAOffset  OutDataTypeStr=uint16
  Constant1 : Constant  Value=inverter.CtSensBOffset  OutDataTypeStr=uint16
  Data Type Conversion : DataTypeConversion  OutDataTypeStr=int32  ConvertRealWorld=Stored Integer (SI)  RndMeth=Simplest
  Data Type Conversion1 : DataTypeConversion  OutDataTypeStr=dataType  RndMeth=Simplest
  Data Type Conversion3 : DataTypeConversion  OutDataTypeStr=fixdt(1,32,17)  ConvertRealWorld=Stored Integer (SI)  RndMeth=Simplest
  Mux : Mux  Inputs=2
  Mux1 : Mux  Inputs=2
  Q17 per unit conversion : ArithShift  BitShiftNumber=-6
  Iab_meas_PU : Outport  VectorParamsAs1DForOutWhenUnconnected=off
  wires:
  Q17 per unit conversion/1 -> Data Type Conversion3/1
  Data Type Conversion/1 -> Add/2
  Add/1 -> Q17 per unit conversion/1
  Data Type Conversion3/1 -> Data Type Conversion1/1
  Data Type Conversion1/1 -> Iab_meas_PU/1
  Ia_ADC/1 -> Mux/1
  Ib_ADC/1 -> Mux/2
  Mux/1 -> Data Type Conversion/1
  Constant/1 -> Mux1/1
  Constant1/1 -> Mux1/2
  Mux1/1 -> Add/1

== system Test_mcb_pmsm_foc_sim_RL/Inverter and Motor - Plant Model/Sensor_Measurements/Get_PU  ==
  rad : Inport
  Constant2 : Constant  Value=2*pi  OutDataTypeStr=single  SampleTime=-1
  Get_PU : Gain  Gain=1/(2*pi)  RndMeth=Simplest  OutDataTypeStr=Inherit: Same as input
  Mod : Math  Operator=mod  SaturateOnIntegerOverflow=on
  PU : Outport  VectorParamsAs1DForOutWhenUnconnected=off
  wires:
  rad/1 -> Mod/1
  Constant2/1 -> Mod/2
  Mod/1 -> Get_PU/1
  Get_PU/1 -> PU/1

== system Test_mcb_pmsm_foc_sim_RL/Inverter and Motor - Plant Model/Sensor_Measurements/Wrap ==
  in : Inport
  Constant2 : Constant  OutDataTypeStr=single  SampleTime=-1
  Mod : Math  Operator=mod  SaturateOnIntegerOverflow=on
  out : Outport  VectorParamsAs1DForOutWhenUnconnected=off
  wires:
  in/1 -> Mod/1
  Constant2/1 -> Mod/2
  Mod/1 -> out/1

== system Test_mcb_pmsm_foc_sim_RL/Inverter and Motor - Plant Model1/Sensor_Measurements/Get_PU  ==
  rad : Inport
  Constant2 : Constant  Value=2*pi  OutDataTypeStr=single  SampleTime=-1
  Get_PU : Gain  Gain=1/(2*pi)  RndMeth=Simplest  OutDataTypeStr=Inherit: Same as input
  Mod : Math  Operator=mod  SaturateOnIntegerOverflow=on
  PU : Outport  VectorParamsAs1DForOutWhenUnconnected=off
  wires:
  rad/1 -> Mod/1
  Constant2/1 -> Mod/2
  Mod/1 -> Get_PU/1
  Get_PU/1 -> PU/1

== system Test_mcb_pmsm_foc_sim_RL/Inverter and Motor - Plant Model1/Sensor_Measurements/Wrap ==
  in : Inport
  Constant2 : Constant  OutDataTypeStr=single  SampleTime=-1
  Mod : Math  Operator=mod  SaturateOnIntegerOverflow=on
  out : Outport  VectorParamsAs1DForOutWhenUnconnected=off
  wires:
  in/1 -> Mod/1
  Constant2/1 -> Mod/2
  Mod/1 -> out/1

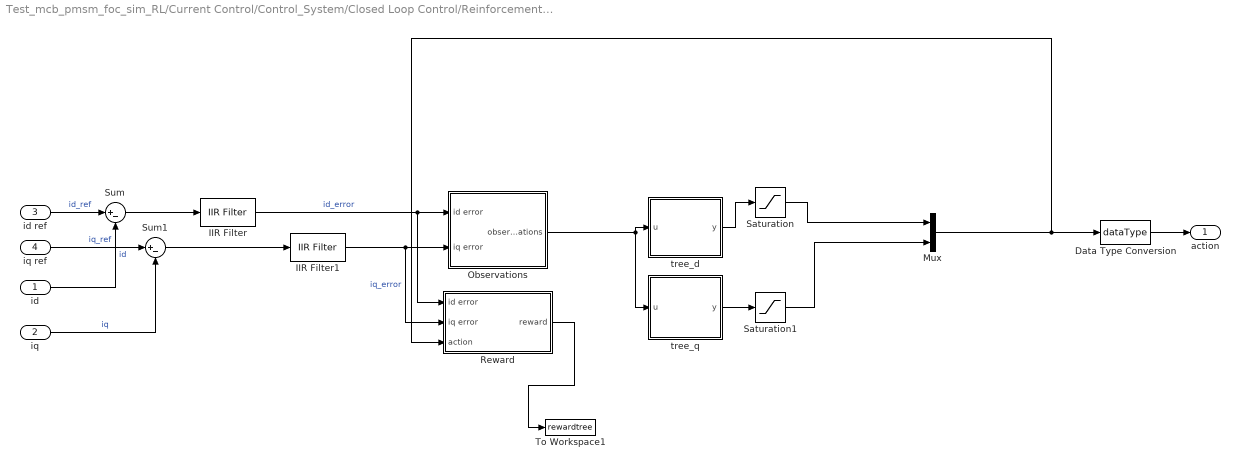
== system Test_mcb_pmsm_foc_sim_RL/Current Control/Control_System/Closed Loop Control/Reinforcement Learning ==
  id : Inport
  iq : Inport  Port=2
  id ref : Inport  Port=3
  iq ref : Inport  Port=4
  Data Type Conversion : DataTypeConversion  OutDataTypeStr=dataType
  IIR Filter : mcbcontrolslib/IIR Filter  Filter_constant=1/200
      settings: SourceProductBaseCode=MT
  IIR Filter1 : mcbcontrolslib/IIR Filter  Filter_constant=1/200
      settings: SourceProductBaseCode=MT
  Mux : Mux  Inputs=2
  Observations : Subsystem
  Reward : Subsystem
  Saturation : Saturate  UpperLimit=1  LowerLimit=-1
  Saturation1 : Saturate  UpperLimit=1  LowerLimit=-1
  Sum : Sum  Inputs=|+-
  Sum1 : Sum  Inputs=|+-
  To Workspace1 : ToWorkspace  VariableName=rewardtree  SampleTime=-1
      settings: Save2DSignal=2-D array (concatenate along first dimension)
  tree_d : MATLAB Function  TreatAsAtomicUnit=on
  tree_q : MATLAB Function  TreatAsAtomicUnit=on
  action : Outport
  wires:
  id ref/1 -> Sum/1  "id_ref"
  id/1 -> Sum/2  "id"
  iq ref/1 -> Sum1/1  "iq_ref"
  iq/1 -> Sum1/2  "iq"
  IIR Filter/1 -> Reward/1(id error), Observations/1(id error)  "id_error"
  IIR Filter1/1 -> Observations/2(iq error), Reward/2(iq error)  "iq_error"
  Observations/1(observations) -> tree_q/1(u), tree_d/1(u)
  Reward/1(reward) -> To Workspace1/1
  Data Type Conversion/1 -> action/1
  Sum/1 -> IIR Filter/1
  Sum1/1 -> IIR Filter1/1
  tree_d/1(y) -> Saturation/1
  tree_q/1(y) -> Saturation1/1
  Saturation/1 -> Mux/1
  Saturation1/1 -> Mux/2
  Mux/1 -> Reward/3(action), Data Type Conversion/1

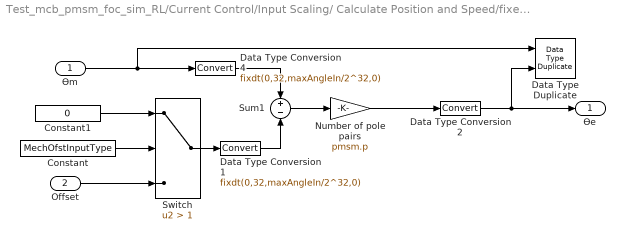
== system Test_mcb_pmsm_foc_sim_RL/Current Control/Input Scaling/ Calculate Position and Speed/fixed-point ==
  ϴm : Inport  OutMin=0  OutMax=maxAngleIn
  Offset : Inport  Port=2
  Constant : Constant  Value=MechOfstInputType  OutDataTypeStr=uint8
  Constant1 : Constant  Value=0  OutDataTypeStr=Inherit: Inherit via back propagation
  Data Type Duplicate : DataTypeDuplicate
  Data Type Conversion1 : DataTypeConversion  OutDataTypeStr=fixdt(0,32,maxAngleIn/2^32,0)  RndMeth=Simplest
  Data Type Conversion2 : DataTypeConversion  OutMin=0  OutMax=maxAngleIn  RndMeth=Simplest
  Data Type Conversion4 : DataTypeConversion  OutDataTypeStr=fixdt(0,32,maxAngleIn/2^32,0)  RndMeth=Simplest
  Number of pole pairs : Gain  Gain=pmsm.p  RndMeth=Simplest  OutDataTypeStr=Inherit: Same as input
  Sum1 : Sum  Inputs=+-  RndMeth=Simplest  OutDataTypeStr=Inherit: Same as first input
  Switch : Switch  Criteria=u2 > Threshold  Threshold=1  OutDataTypeStr=Inherit: Inherit via back propagation
  ϴe : Outport  VectorParamsAs1DForOutWhenUnconnected=off
  wires:
  Constant1/1 -> Switch/1
  Data Type Conversion1/1 -> Sum1/2
  Constant/1 -> Switch/2
  ϴm/1 -> Data Type Conversion4/1, Data Type Duplicate/1
  Switch/1 -> Data Type Conversion1/1
  Number of pole pairs/1 -> Data Type Conversion2/1
  Data Type Conversion2/1 -> Data Type Duplicate/2, ϴe/1
  Sum1/1 -> Number of pole pairs/1
  Data Type Conversion4/1 -> Sum1/1
  Offset/1 -> Switch/3

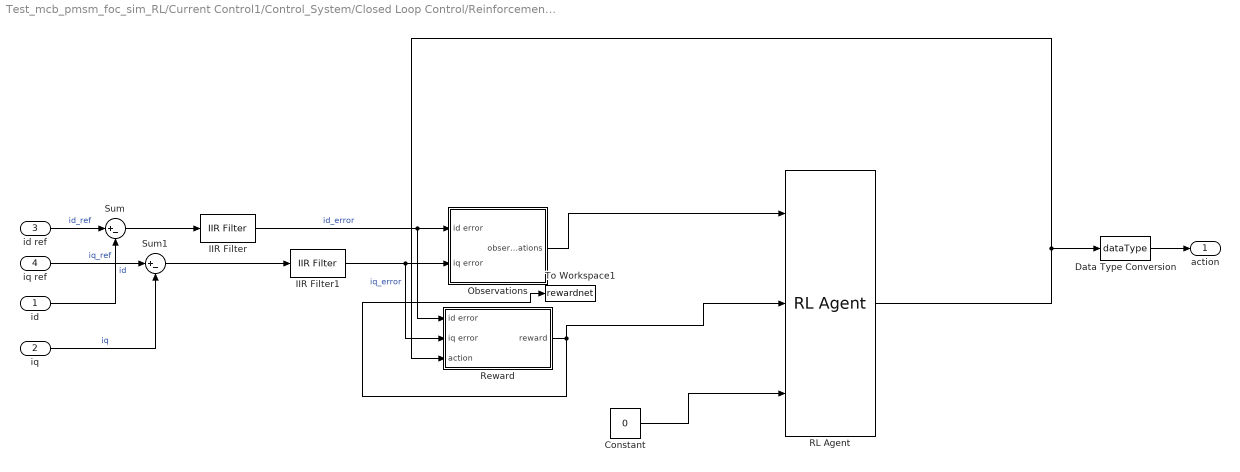
== system Test_mcb_pmsm_foc_sim_RL/Current Control1/Control_System/Closed Loop Control/Reinforcement Learning ==
  id : Inport
  iq : Inport  Port=2
  id ref : Inport  Port=3
  iq ref : Inport  Port=4
  Constant : Constant  Value=0
  Data Type Conversion : DataTypeConversion  OutDataTypeStr=dataType
  IIR Filter : mcbcontrolslib/IIR Filter  Filter_constant=1/200
      settings: SourceProductBaseCode=MT
  IIR Filter1 : mcbcontrolslib/IIR Filter  Filter_constant=1/200
      settings: SourceProductBaseCode=MT
  Observations : Subsystem
  RL Agent : rllib/RL Agent  Agent=agent  ProvideReward=on  ProvideIsDone=on  ProvideCumRwd=off  TreatAsDirectFeedthrough=on  CollectLoggedSignals=on  CollectModelStates=on
      settings: SourceProductName=Reinforcement Learning
  Reward : Subsystem
  Sum : Sum  Inputs=|+-
  Sum1 : Sum  Inputs=|+-
  To Workspace1 : ToWorkspace  VariableName=rewardnet  SampleTime=-1
      settings: Save2DSignal=2-D array (concatenate along first dimension)
  action : Outport
  wires:
  id ref/1 -> Sum/1  "id_ref"
  id/1 -> Sum/2  "id"
  iq ref/1 -> Sum1/1  "iq_ref"
  iq/1 -> Sum1/2  "iq"
  IIR Filter/1 -> Reward/1(id error), Observations/1(id error)  "id_error"
  IIR Filter1/1 -> Observations/2(iq error), Reward/2(iq error)  "iq_error"
  Observations/1(observations) -> RL Agent/1
  Reward/1(reward) -> To Workspace1/1, RL Agent/2
  Data Type Conversion/1 -> action/1
  Sum/1 -> IIR Filter/1
  Sum1/1 -> IIR Filter1/1
  Constant/1 -> RL Agent/3
  RL Agent/1 -> Reward/3(action), Data Type Conversion/1

== system Test_mcb_pmsm_foc_sim_RL/Current Control1/Input Scaling/ Calculate Position and Speed/fixed-point ==
  ϴm : Inport  OutMin=0  OutMax=maxAngleIn
  Offset : Inport  Port=2
  Constant : Constant  Value=MechOfstInputType  OutDataTypeStr=uint8
  Constant1 : Constant  Value=0  OutDataTypeStr=Inherit: Inherit via back propagation
  Data Type Duplicate : DataTypeDuplicate
  Data Type Conversion1 : DataTypeConversion  OutDataTypeStr=fixdt(0,32,maxAngleIn/2^32,0)  RndMeth=Simplest
  Data Type Conversion2 : DataTypeConversion  OutMin=0  OutMax=maxAngleIn  RndMeth=Simplest
  Data Type Conversion4 : DataTypeConversion  OutDataTypeStr=fixdt(0,32,maxAngleIn/2^32,0)  RndMeth=Simplest
  Number of pole pairs : Gain  Gain=pmsm.p  RndMeth=Simplest  OutDataTypeStr=Inherit: Same as input
  Sum1 : Sum  Inputs=+-  RndMeth=Simplest  OutDataTypeStr=Inherit: Same as first input
  Switch : Switch  Criteria=u2 > Threshold  Threshold=1  OutDataTypeStr=Inherit: Inherit via back propagation
  ϴe : Outport  VectorParamsAs1DForOutWhenUnconnected=off
  wires:
  Constant1/1 -> Switch/1
  Data Type Conversion1/1 -> Sum1/2
  Constant/1 -> Switch/2
  ϴm/1 -> Data Type Conversion4/1, Data Type Duplicate/1
  Switch/1 -> Data Type Conversion1/1
  Number of pole pairs/1 -> Data Type Conversion2/1
  Data Type Conversion2/1 -> Data Type Duplicate/2, ϴe/1
  Sum1/1 -> Number of pole pairs/1
  Data Type Conversion4/1 -> Sum1/1
  Offset/1 -> Switch/3

== system Test_mcb_pmsm_foc_sim_RL/Current Control/Control_System/Closed Loop Control/Reinforcement Learning/Observations ==
  id error : Inport
  iq error : Inport  Port=2
  Discrete Derivative : simulink/Discrete/Discrete Derivative  gainval=1  ICPrevScaledInput=0.0  OutMin=[]  OutMax=[]  OutDataTypeStr=Inherit: Inherit via back propagation  OutDataType=fixdt(1, 16)  OutScaling=2^-10  DoSatur=off
  Discrete Derivative1 : simulink/Discrete/Discrete Derivative  gainval=1  ICPrevScaledInput=0.0  OutMin=[]  OutMax=[]  OutDataTypeStr=Inherit: Inherit via back propagation  OutDataType=fixdt(1, 16)  OutScaling=2^-10  DoSatur=off
  Discrete-Time Integrator : DiscreteIntegrator  SampleTime=-1  OutDataTypeStr=Inherit: Inherit via back propagation  SaturateOnIntegerOverflow=on  UpperSaturationLimit=1  LowerSaturationLimit=-1  ICPrevOutput=DiscIntNeverNeededParam  ICPrevScaledInput=DiscIntNeverNeededParam
  Discrete-Time Integrator1 : DiscreteIntegrator  SampleTime=-1  OutDataTypeStr=Inherit: Inherit via back propagation  SaturateOnIntegerOverflow=on  ICPrevOutput=DiscIntNeverNeededParam  ICPrevScaledInput=DiscIntNeverNeededParam
  Gain : Gain  Gain=1e-5  OutDataTypeStr=Inherit: Same as input
  Gain1 : Gain  Gain=1e-5  OutDataTypeStr=Inherit: Same as input
  Gain2 : Gain  Gain=0.5  OutDataTypeStr=Inherit: Same as input
  Gain3 : Gain  Gain=0.5  OutDataTypeStr=Inherit: Same as input
  Mux1 : Mux  Inputs=6
  observations : Outport  VectorParamsAs1DForOutWhenUnconnected=off
  wires:
  Discrete Derivative/1 -> Gain/1
  Discrete Derivative1/1 -> Gain1/1
  Discrete-Time Integrator/1 -> Mux1/5  "integral e_id"
  Discrete-Time Integrator1/1 -> Mux1/6  "integral e_iq"
  Mux1/1 -> observations/1
  Gain/1 -> Mux1/3  "deriv e_id"
  Gain1/1 -> Mux1/4  "deriv e_iq"
  id error/1 -> Discrete-Time Integrator/1, Discrete Derivative/1, Gain2/1  "e_id"
  iq error/1 -> Discrete-Time Integrator1/1, Discrete Derivative1/1, Gain3/1  "e_iq"
  Gain2/1 -> Mux1/1
  Gain3/1 -> Mux1/2

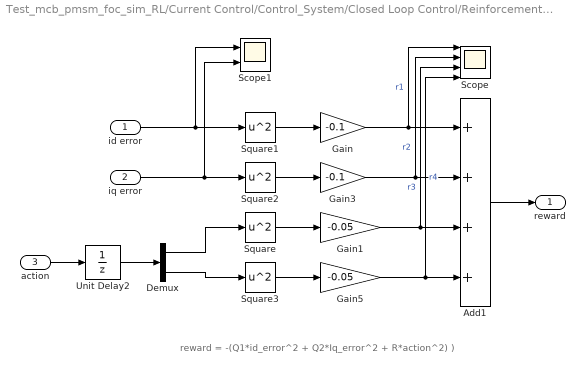
== system Test_mcb_pmsm_foc_sim_RL/Current Control/Control_System/Closed Loop Control/Reinforcement Learning/Reward ==
  note: reward = -(Q1*id_error^2 + Q2*Iq_error^2 + R*action^2) )
  id error : Inport
  iq error : Inport  Port=2
  action : Inport  Port=3
  Add1 : Sum  Inputs=++++
  Demux : Demux  Outputs=2
  Gain : Gain  Gain=-0.1
  Gain1 : Gain  Gain=-0.05
  Gain3 : Gain  Gain=-0.1
  Gain5 : Gain  Gain=-0.05
  Scope : Scope  NumInputPorts=4
  Scope1 : Scope  NumInputPorts=2
  Square{,1..3} (4 alike) : Math  Operator=square  SaturateOnIntegerOverflow=on
  Unit Delay2 : UnitDelay  SampleTime=-1  HasFrameUpgradeWarning=on
  reward : Outport  VectorParamsAs1DForOutWhenUnconnected=off
  wires:
  Square1/1 -> Gain/1
  Square2/1 -> Gain3/1
  Demux/1 -> Square/1
  Square/1 -> Gain1/1
  Gain1/1 -> Scope/3, Add1/3  "r3"
  Demux/2 -> Square3/1
  Square3/1 -> Gain5/1
  Unit Delay2/1 -> Demux/1
  action/1 -> Unit Delay2/1
  Add1/1 -> reward/1
  Gain5/1 -> Scope/4, Add1/4  "r4"
  Gain/1 -> Add1/1, Scope/1  "r1"
  Gain3/1 -> Scope/2, Add1/2  "r2"
  id error/1 -> Square1/1, Scope1/1
  iq error/1 -> Square2/1, Scope1/2

== system Test_mcb_pmsm_foc_sim_RL/Current Control1/Control_System/Closed Loop Control/Reinforcement Learning/Observations ==
  id error : Inport
  iq error : Inport  Port=2
  Discrete Derivative : simulink/Discrete/Discrete Derivative  gainval=1  ICPrevScaledInput=0.0  OutMin=[]  OutMax=[]  OutDataTypeStr=Inherit: Inherit via back propagation  OutDataType=fixdt(1, 16)  OutScaling=2^-10  DoSatur=off
  Discrete Derivative1 : simulink/Discrete/Discrete Derivative  gainval=1  ICPrevScaledInput=0.0  OutMin=[]  OutMax=[]  OutDataTypeStr=Inherit: Inherit via back propagation  OutDataType=fixdt(1, 16)  OutScaling=2^-10  DoSatur=off
  Discrete-Time Integrator : DiscreteIntegrator  SampleTime=-1  OutDataTypeStr=Inherit: Inherit via back propagation  SaturateOnIntegerOverflow=on  UpperSaturationLimit=1  LowerSaturationLimit=-1  ICPrevOutput=DiscIntNeverNeededParam  ICPrevScaledInput=DiscIntNeverNeededParam
  Discrete-Time Integrator1 : DiscreteIntegrator  SampleTime=-1  OutDataTypeStr=Inherit: Inherit via back propagation  SaturateOnIntegerOverflow=on  ICPrevOutput=DiscIntNeverNeededParam  ICPrevScaledInput=DiscIntNeverNeededParam
  Gain : Gain  Gain=1e-5  OutDataTypeStr=Inherit: Same as input
  Gain1 : Gain  Gain=1e-5  OutDataTypeStr=Inherit: Same as input
  Gain2 : Gain  Gain=0.5  OutDataTypeStr=Inherit: Same as input
  Gain3 : Gain  Gain=0.5  OutDataTypeStr=Inherit: Same as input
  Mux1 : Mux  Inputs=6
  observations : Outport  VectorParamsAs1DForOutWhenUnconnected=off
  wires:
  Discrete Derivative/1 -> Gain/1
  Discrete Derivative1/1 -> Gain1/1
  Discrete-Time Integrator/1 -> Mux1/5  "integral e_id"
  Discrete-Time Integrator1/1 -> Mux1/6  "integral e_iq"
  Mux1/1 -> observations/1
  Gain/1 -> Mux1/3  "deriv e_id"
  Gain1/1 -> Mux1/4  "deriv e_iq"
  id error/1 -> Discrete-Time Integrator/1, Discrete Derivative/1, Gain2/1  "e_id"
  iq error/1 -> Discrete-Time Integrator1/1, Discrete Derivative1/1, Gain3/1  "e_iq"
  Gain2/1 -> Mux1/1
  Gain3/1 -> Mux1/2

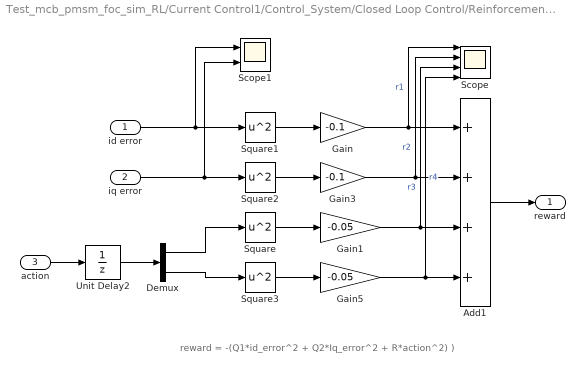
== system Test_mcb_pmsm_foc_sim_RL/Current Control1/Control_System/Closed Loop Control/Reinforcement Learning/Reward ==
  note: reward = -(Q1*id_error^2 + Q2*Iq_error^2 + R*action^2) )
  id error : Inport
  iq error : Inport  Port=2
  action : Inport  Port=3
  Add1 : Sum  Inputs=++++
  Demux : Demux  Outputs=2
  Gain : Gain  Gain=-0.1
  Gain1 : Gain  Gain=-0.05
  Gain3 : Gain  Gain=-0.1
  Gain5 : Gain  Gain=-0.05
  Scope : Scope  NumInputPorts=4
  Scope1 : Scope  NumInputPorts=2
  Square{,1..3} (4 alike) : Math  Operator=square  SaturateOnIntegerOverflow=on
  Unit Delay2 : UnitDelay  SampleTime=-1  HasFrameUpgradeWarning=on
  reward : Outport  VectorParamsAs1DForOutWhenUnconnected=off
  wires:
  Square1/1 -> Gain/1
  Square2/1 -> Gain3/1
  Demux/1 -> Square/1
  Square/1 -> Gain1/1
  Gain1/1 -> Scope/3, Add1/3  "r3"
  Demux/2 -> Square3/1
  Square3/1 -> Gain5/1
  Unit Delay2/1 -> Demux/1
  action/1 -> Unit Delay2/1
  Add1/1 -> reward/1
  Gain5/1 -> Scope/4, Add1/4  "r4"
  Gain/1 -> Add1/1, Scope/1  "r1"
  Gain3/1 -> Scope/2, Add1/2  "r2"
  id error/1 -> Square1/1, Scope1/1
  iq error/1 -> Square2/1, Scope1/2
